simulink model "s3"  (R2016b)
settings: Solver=VariableStepAuto  StartTime=0.0  StopTime=10.0  RelTol=1e-3
settings Model: Creator=fabia  LastModifiedBy=fabia

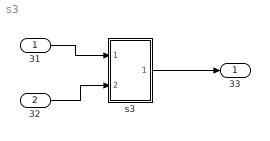
== system s3 ==
  31 : Inport
  32 : Inport  Port=2
  s3 : Subsystem
  33 : Outport
  wires:
  31/1 -> s3/1(In1)
  32/1 -> s3/2(In2)
  s3/1(Out1) -> 33/1

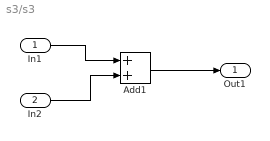
== system s3/s3 ==
  In1 : Inport
  In2 : Inport  Port=2
  Add1 : Sum
  Out1 : Outport
  wires:
  Add1/1 -> Out1/1
  In1/1 -> Add1/1
  In2/1 -> Add1/2
